simulink model "IEEE24bus"  (R2019b)
settings: Solver=VariableStepAuto  StartTime=0.0  StopTime=100  RelTol=1e-3
values from neighbouring files (symbols this model uses):
  C_b = 1/(w_b*Z_b)    (= 5.01433343075e-06)    [IEEE24_bus.m]
  Exc = [ 011	0	 200	0.02	1.12   0.5   0	0       0       0       0       0 ... (first row only)    [IEEE24_bus.m]
  G_data = [ 011	15.8 138	2.8	0.2     2.7	1.5     0.3     7.5     0.25	0.04	0.85	0.85	0.25	0.12	0 ... (first row only)    [IEEE24_bus.m]
  H011 = 4    [IEEE24_bus.m]
  H012 = 4    [IEEE24_bus.m]
  H013 = 4    [IEEE24_bus.m]
  H021 = 4    [IEEE24_bus.m]
  H022 = 4    [IEEE24_bus.m]
  H023 = 4    [IEEE24_bus.m]
  H024 = 4    [IEEE24_bus.m]
  H025 = 4    [IEEE24_bus.m]
  H026 = 4    [IEEE24_bus.m]
  H131 = 4    [IEEE24_bus.m]
  H132 = 4    [IEEE24_bus.m]
  H133 = 4    [IEEE24_bus.m]
  H134 = 4    [IEEE24_bus.m]
  H135 = 4    [IEEE24_bus.m]
  H151 = 4    [IEEE24_bus.m]
  H152 = 4    [IEEE24_bus.m]
  H153 = 4    [IEEE24_bus.m]
  H154 = 4    [IEEE24_bus.m]
  H161 = 4    [IEEE24_bus.m]
  H181 = 3.25    [IEEE24_bus.m]
  H211 = 4    [IEEE24_bus.m]
  H212 = 4    [IEEE24_bus.m]
  H213 = 4    [IEEE24_bus.m]
  H215 = 4    [IEEE24_bus.m]
  H216 = 4    [IEEE24_bus.m]
  H221 = 3.25    [IEEE24_bus.m]
  H231 = 4    [IEEE24_bus.m]
  H232 = 4    [IEEE24_bus.m]
  H233 = 4    [IEEE24_bus.m]
  H234 = 4    [IEEE24_bus.m]
  H235 = 4    [IEEE24_bus.m]
  L_b = Z_b/w_b    (= 1.40321608159)    [IEEE24_bus.m]
  PSSMODEL = 1    [IEEE24_bus.m]    (also in IEEE24bus_simplified_benchmark.m)
  Z_b = (V_b^2)/S_b    (= 529)    [IEEE24_bus.m]
undefined symbols (not defined in the file or in its folder): D1, Delta
libraries: powerlib x258, sps_avr x33, microgridLibrary x6
(part 3 of 6)

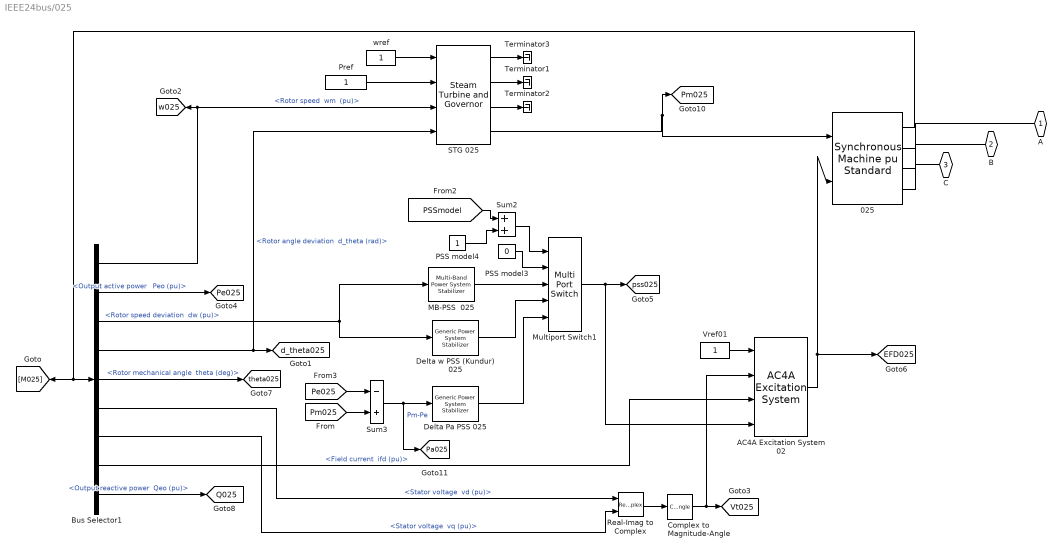
== system IEEE24bus/025 ==
  025 : powerlib/Machines/Synchronous Machine pu Standard  PresetModel=No  MechanicalLoad=Mechanical power Pm  ShowDetailedParameters=on  RotorType=Round  Units=per unit standard parameters  MeasurementBus=off  NominalParameters="[G_data(8,2)*1E6  G_data(8,3)*1E3  60]"  Reactances1=[G_data(8,6),G_data(8,8),G_data(8,10),G_data(8,7),G_data(8,12),G_data(8,14),G_data(8,5)]  Reactances2=[G_data(6,6),G_data(6,8),G_data(6,10),G_data(6,7),G_data(6,12),G_data(6,14),G_data(6,5)]  dAxisTimeConstants=Open-circuit  qAxisTimeConstants=Open-circuit  TimeConstants1="[G_data(6,9)  G_data(6,11)  G_data(6,13)  G_data(6,15)]"  TimeConstants2="[G_data(8,9)  G_data(8,11)  G_data(8,13)  G_data(8,15)]"  TimeConstants3="[  5.9  0.033  0.023  ]"  TimeConstants4=[ 8.0, 0.03, 0.3371, 0.0295 ]  TimeConstants5=[ 1.01, 0.053, 0.1 ]  TimeConstants6=[ 1.3201, 0.023, 1.0, 0.07 ]  TimeConstants7="[  1.01  0.053  0.051266  ]"  TimeConstants8=[ 1.3201, 0.0231, 0.3371, 0.0295 ]  StatorResistance=0  Mechanical="[ H025 0  4 ]"  PolePairs=4  InitialConditions=[0 -49.0871 0.832503 0.832503 0.832503 -10.6328 -130.633 109.367 2.39024]  SetSaturation=off  Saturation=[0.6404,0.7127,0.8441,0.9214,0.9956,1.082,1.19,1.316,1.457;0.7,0.7698,0.8872,0.9466,0.9969,1.046,1.1,1.151,1.201]  LoadFlowParameters=[1 3330000000 20000 0 0]  TsPowergui=0  TsBlock=-1  IterativeModel=Forward Euler  IterativeDiscreteModel=Trapezoidal non iterative  BusType=PV  Pref=G_data(8,2)*1e6  Qref=0  Qmin=-inf  Qmax=inf  PLF=0  QLF=0
      settings: SourceProductName=Simscape Power Systems
  AC4A Excitation System 02 : sps_avr/AC4A Excitation System  Tr=Exc(1,2)  KaTa="[Exc(1,3)   Exc(1,4)]"  VIminmax=[-10 10]  VRminmax=[-4.53 5.64]  TbTc="[Exc(1,5)  Exc(1,6)]"  Kc=0  v0=[1 2.3902]  TsBlock=0
      settings: SourceProductName=Simscape Power Systems  SourceProductBaseCode=PS
  Bus Selector1 : BusSelector  OutputSignals="Mechanical.Rotor speed  wm  (pu),Output active power   Peo (pu),Mechanical.Rotor speed deviation  dw (pu),Mechanical.Rotor angle deviation  d_theta (rad),Mechanical.Rotor mechanical angle  theta (deg),dq0 components.Stator voltage  vd (pu),dq0 components.Stator voltage  vq (pu),dq0 components.Field current  ifd (pu),Output reactive power  Qeo (pu)"
  Complex to Magnitude-Angle : ComplexToMagnitudeAngle  Output=Magnitude
  "Delta Pa PSS 025 " : powerlib/Machines/Generic Power System Stabilizer  Tsensor=15e-3  K=2.5*1.25  Twashout=1  Tleadlag1=[60e-3 1]  Tleadlag2=[0 0]  VSlimits=[-0.15 0.15]  Vinit=0  Plot_On=off  MagdB_On=on  FreqRange=logspace(-2,2,500)
      settings: SourceProductName=Simscape Power Systems  SourceProductBaseCode=PS
  "Delta w PSS (Kundur) 025 " : powerlib/Machines/Generic Power System Stabilizer  Tsensor=15e-3  K=30  Twashout=10  Tleadlag1=[50e-3 20e-3]  Tleadlag2=[3 5.4]  VSlimits=[-0.15 0.15]  Vinit=0  Plot_On=off  MagdB_On=on  FreqRange=logspace(-2,2,500)
      settings: SourceProductName=Simscape Power Systems  SourceProductBaseCode=PS
  MB-PSS  025 : powerlib/Machines/Multi-Band Power System Stabilizer  OperationMode=Simplified settings  Kg=1  GL=[0.1 10]  GI="[1  10]"  GH="[13  120]"  GLd=[66 66 9.4]  TcLF=[1.667 2 0 0 0 0 2 2.4 0 0 0 0 1 1]  GId=[66 66 47.6]  TcIF=[1 1 0.25 0.3 0 0 1 1 0.3 0.36 0 0 0 0]  GHd=[66 66 233]  TcHF="[0.01 0.012 0 0 0 0  0.012 0.0144 0 0 0 0 1 1]"  LIM=[.075 .15 .15 .15]  Plot_On=off  MagdB_On=off  FreqRange=logspace(-2,2,500)
      settings: SourceProductName=Simscape Power Systems  SourceProductBaseCode=PS
  Multiport Switch1 : MultiPortSwitch  Inputs=4  InputSameDT=on
  PSS model3 : Constant  Value=0
  PSS model4 : Constant
  Pref : Constant
  Real-Imag to Complex : RealImagToComplex
  STG 025 : powerlib/Machines/Steam Turbine and Governor  gentype=Tandem-compound (single mass)  reg1="[ 1  0.05    0 ]"  reg2="[ 0.001  0.15 ]"  reg3="[ -0.1  0.1  0  4.496 ]"  N=3600  turb1="[ 0  10   3.3   0.5   ]"  turb2="[   0   0.36    0.36   0.28   ]"  HA="[ 0.046  1.430  1.465   0.192 ]"  KA="[ 90.44  53.88  64.59   62.94  ]"  DA="[ 0.0115  0.3575  0.3663   0.0137  ]"  ini1=1  ini2=[0.779316,-31.4247]
      settings: SourceProductName=Simscape Power Systems  SourceProductBaseCode=PS
  Sum2 : Sum  SaturateOnIntegerOverflow=on  InputSameDT=on  OutDataTypeStr=Inherit: Same as first input
  Sum3 : Sum  Inputs=-+  SaturateOnIntegerOverflow=on  InputSameDT=on  OutDataTypeStr=Inherit: Same as first input
  Terminator1 : Terminator
  Terminator2 : Terminator
  Terminator3 : Terminator
  Vref01 : Constant
  wref : Constant
  A : PMIOPort  Side=Left
  B : PMIOPort  Port=2  Side=Left
  C : PMIOPort  Port=3  Side=Left
  tag scope: EFD025=global, Pa025=global, Pe025=global, Pm025=global, Q025=global, Vt025=global, d_theta025=global, pss025=global, theta025=global, w025=global
  wires:
  Bus Selector1/7 -> Real-Imag to Complex/2  "<Stator voltage  vq (pu)>"
  Bus Selector1/6 -> Real-Imag to Complex/1  "<Stator voltage  vd (pu)>"
  wref/1 -> STG 025/1
  Vref01/1 -> AC4A Excitation System 02/1
  Bus Selector1/4 -> [d_theta025], STG 025/4  "<Rotor angle deviation  d_theta (rad)>"
  025/1 -> Bus Selector1/1, [M025]
  Bus Selector1/1 -> [w025], STG 025/3  "<Rotor speed  wm  (pu)>"
  Bus Selector1/3 -> "Delta w PSS (Kundur) 025 "/1, MB-PSS  025/1  "<Rotor speed deviation  dw (pu)>"
  Real-Imag to Complex/1 -> Complex to Magnitude-Angle/1
  Complex to Magnitude-Angle/1 -> AC4A Excitation System 02/2, [Vt025]
  AC4A Excitation System 02/1 -> 025/2, [EFD025]
  Multiport Switch1/1 -> AC4A Excitation System 02/4, [pss025]
  Bus Selector1/5 -> [theta025]  "<Rotor mechanical angle  theta (deg)>"
  Bus Selector1/2 -> [Pe025]  "<Output active power   Peo (pu)>"
  Bus Selector1/8 -> AC4A Excitation System 02/3  "<Field current  ifd (pu)>"
  STG 025/4 -> [Pm025], 025/1
  Pref/1 -> STG 025/2
  Bus Selector1/9 -> [Q025]  "<Output reactive power  Qeo (pu)>"
  PSS model4/1 -> Sum2/2
  Sum2/1 -> Multiport Switch1/1
  [PSSmodel] -> Sum2/1
  PSS model3/1 -> Multiport Switch1/2
  Sum3/1 -> [Pa025], "Delta Pa PSS 025 "/1  "Pm-Pe"
  "Delta Pa PSS 025 "/1 -> Multiport Switch1/5
  "Delta w PSS (Kundur) 025 "/1 -> Multiport Switch1/4
  [Pm025] -> Sum3/2
  [Pe025] -> Sum3/1
  MB-PSS  025/1 -> Multiport Switch1/3
  STG 025/1 -> Terminator3/1
  STG 025/2 -> Terminator1/1
  STG 025/3 -> Terminator2/1
  connections:
  025/RConn1 -- A/RConn1
  025/RConn2 -- B/RConn1
  025/RConn3 -- C/RConn1

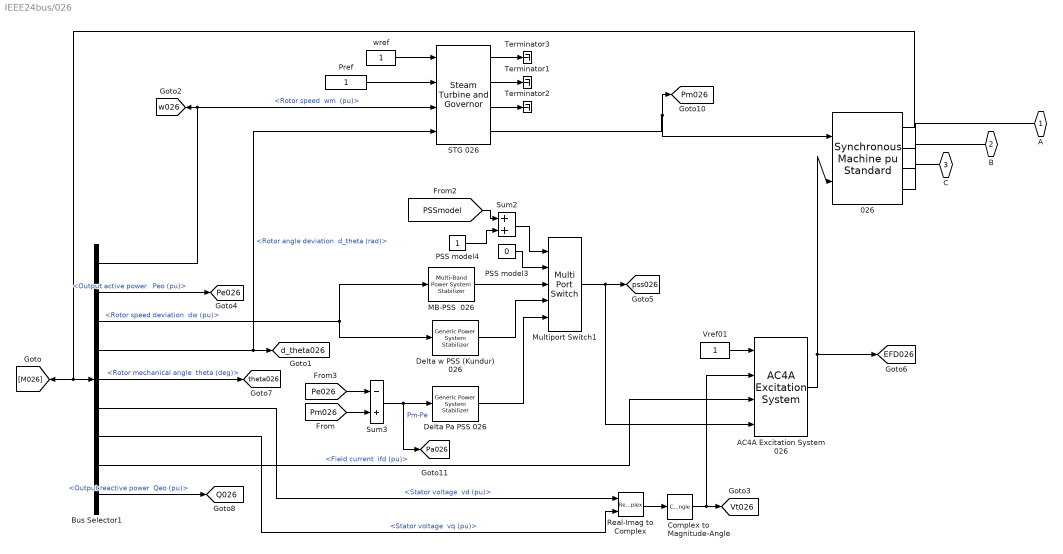
== system IEEE24bus/026 ==
  026 : powerlib/Machines/Synchronous Machine pu Standard  PresetModel=No  MechanicalLoad=Mechanical power Pm  ShowDetailedParameters=on  RotorType=Round  Units=per unit standard parameters  MeasurementBus=off  NominalParameters="[G_data(9,2)*1E6  G_data(9,3)*1E3  60]"  Reactances1=[G_data(9,6),G_data(9,8),G_data(9,10),G_data(9,7),G_data(9,12),G_data(9,14),G_data(9,5)]  Reactances2=[G_data(6,6),G_data(6,8),G_data(6,10),G_data(6,7),G_data(6,12),G_data(6,14),G_data(6,5)]  dAxisTimeConstants=Open-circuit  qAxisTimeConstants=Open-circuit  TimeConstants1="[G_data(6,9)  G_data(6,11)  G_data(6,13)  G_data(6,15)]"  TimeConstants2="[G_data(9,9)  G_data(9,11)  G_data(9,13)  G_data(9,15)]"  TimeConstants3="[  5.9  0.033  0.023  ]"  TimeConstants4=[ 8.0, 0.03, 0.3371, 0.0295 ]  TimeConstants5=[ 1.01, 0.053, 0.1 ]  TimeConstants6=[ 1.3201, 0.023, 1.0, 0.07 ]  TimeConstants7="[  1.01  0.053  0.051266  ]"  TimeConstants8=[ 1.3201, 0.0231, 0.3371, 0.0295 ]  StatorResistance=0  Mechanical="[ H026 0  4 ]"  PolePairs=4  InitialConditions=[0 -49.0871 0.832503 0.832503 0.832503 -10.6328 -130.633 109.367 2.39024]  SetSaturation=off  Saturation=[0.6404,0.7127,0.8441,0.9214,0.9956,1.082,1.19,1.316,1.457;0.7,0.7698,0.8872,0.9466,0.9969,1.046,1.1,1.151,1.201]  LoadFlowParameters=[1 3330000000 20000 0 0]  TsPowergui=0  TsBlock=-1  IterativeModel=Forward Euler  IterativeDiscreteModel=Trapezoidal non iterative  BusType=PV  Pref=G_data(9,2)*1e6  Qref=0  Qmin=-inf  Qmax=inf  PLF=0  QLF=0
      settings: SourceProductName=Simscape Power Systems
  AC4A Excitation System 026 : sps_avr/AC4A Excitation System  Tr=Exc(1,2)  KaTa="[Exc(1,3)   Exc(1,4)]"  VIminmax=[-10 10]  VRminmax=[-4.53 5.64]  TbTc="[Exc(1,5)  Exc(1,6)]"  Kc=0  v0=[1 2.3902]  TsBlock=0
      settings: SourceProductName=Simscape Power Systems  SourceProductBaseCode=PS
  Bus Selector1 : BusSelector  OutputSignals="Mechanical.Rotor speed  wm  (pu),Output active power   Peo (pu),Mechanical.Rotor speed deviation  dw (pu),Mechanical.Rotor angle deviation  d_theta (rad),Mechanical.Rotor mechanical angle  theta (deg),dq0 components.Stator voltage  vd (pu),dq0 components.Stator voltage  vq (pu),dq0 components.Field current  ifd (pu),Output reactive power  Qeo (pu)"
  Complex to Magnitude-Angle : ComplexToMagnitudeAngle  Output=Magnitude
  "Delta Pa PSS 026 " : powerlib/Machines/Generic Power System Stabilizer  Tsensor=15e-3  K=2.5*1.25  Twashout=1  Tleadlag1=[60e-3 1]  Tleadlag2=[0 0]  VSlimits=[-0.15 0.15]  Vinit=0  Plot_On=off  MagdB_On=on  FreqRange=logspace(-2,2,500)
      settings: SourceProductName=Simscape Power Systems  SourceProductBaseCode=PS
  "Delta w PSS (Kundur) 026 " : powerlib/Machines/Generic Power System Stabilizer  Tsensor=15e-3  K=30  Twashout=10  Tleadlag1=[50e-3 20e-3]  Tleadlag2=[3 5.4]  VSlimits=[-0.15 0.15]  Vinit=0  Plot_On=off  MagdB_On=on  FreqRange=logspace(-2,2,500)
      settings: SourceProductName=Simscape Power Systems  SourceProductBaseCode=PS
  MB-PSS  026 : powerlib/Machines/Multi-Band Power System Stabilizer  OperationMode=Simplified settings  Kg=1  GL=[0.1 10]  GI="[1  10]"  GH="[13  120]"  GLd=[66 66 9.4]  TcLF=[1.667 2 0 0 0 0 2 2.4 0 0 0 0 1 1]  GId=[66 66 47.6]  TcIF=[1 1 0.25 0.3 0 0 1 1 0.3 0.36 0 0 0 0]  GHd=[66 66 233]  TcHF="[0.01 0.012 0 0 0 0  0.012 0.0144 0 0 0 0 1 1]"  LIM=[.075 .15 .15 .15]  Plot_On=off  MagdB_On=off  FreqRange=logspace(-2,2,500)
      settings: SourceProductName=Simscape Power Systems  SourceProductBaseCode=PS
  Multiport Switch1 : MultiPortSwitch  Inputs=4  InputSameDT=on
  PSS model3 : Constant  Value=0
  PSS model4 : Constant
  Pref : Constant
  Real-Imag to Complex : RealImagToComplex
  STG 026 : powerlib/Machines/Steam Turbine and Governor  gentype=Tandem-compound (single mass)  reg1="[ 1  0.05    0 ]"  reg2="[ 0.001  0.15 ]"  reg3="[ -0.1  0.1  0  4.496 ]"  N=3600  turb1="[ 0  10   3.3   0.5   ]"  turb2="[   0   0.36    0.36   0.28   ]"  HA="[ 0.046  1.430  1.465   0.192 ]"  KA="[ 90.44  53.88  64.59   62.94  ]"  DA="[ 0.0115  0.3575  0.3663   0.0137  ]"  ini1=0.9  ini2=[0.779316,-31.4247]
      settings: SourceProductName=Simscape Power Systems  SourceProductBaseCode=PS
  Sum2 : Sum  SaturateOnIntegerOverflow=on  InputSameDT=on  OutDataTypeStr=Inherit: Same as first input
  Sum3 : Sum  Inputs=-+  SaturateOnIntegerOverflow=on  InputSameDT=on  OutDataTypeStr=Inherit: Same as first input
  Terminator1 : Terminator
  Terminator2 : Terminator
  Terminator3 : Terminator
  Vref01 : Constant
  wref : Constant
  A : PMIOPort  Side=Left
  B : PMIOPort  Port=2  Side=Left
  C : PMIOPort  Port=3  Side=Left
  tag scope: EFD026=global, Pa026=global, Pe026=global, Pm026=global, Q026=global, Vt026=global, d_theta026=global, pss026=global, theta026=global, w026=global
  wires:
  Bus Selector1/7 -> Real-Imag to Complex/2  "<Stator voltage  vq (pu)>"
  Bus Selector1/6 -> Real-Imag to Complex/1  "<Stator voltage  vd (pu)>"
  wref/1 -> STG 026/1
  Vref01/1 -> AC4A Excitation System 026/1
  Bus Selector1/4 -> [d_theta026], STG 026/4  "<Rotor angle deviation  d_theta (rad)>"
  026/1 -> Bus Selector1/1, [M026]
  Bus Selector1/1 -> [w026], STG 026/3  "<Rotor speed  wm  (pu)>"
  Bus Selector1/3 -> "Delta w PSS (Kundur) 026 "/1, MB-PSS  026/1  "<Rotor speed deviation  dw (pu)>"
  Real-Imag to Complex/1 -> Complex to Magnitude-Angle/1
  Complex to Magnitude-Angle/1 -> AC4A Excitation System 026/2, [Vt026]
  AC4A Excitation System 026/1 -> 026/2, [EFD026]
  Multiport Switch1/1 -> AC4A Excitation System 026/4, [pss026]
  Bus Selector1/5 -> [theta026]  "<Rotor mechanical angle  theta (deg)>"
  Bus Selector1/2 -> [Pe026]  "<Output active power   Peo (pu)>"
  Bus Selector1/8 -> AC4A Excitation System 026/3  "<Field current  ifd (pu)>"
  STG 026/4 -> [Pm026], 026/1
  Pref/1 -> STG 026/2
  Bus Selector1/9 -> [Q026]  "<Output reactive power  Qeo (pu)>"
  PSS model4/1 -> Sum2/2
  Sum2/1 -> Multiport Switch1/1
  [PSSmodel] -> Sum2/1
  PSS model3/1 -> Multiport Switch1/2
  Sum3/1 -> [Pa026], "Delta Pa PSS 026 "/1  "Pm-Pe"
  "Delta Pa PSS 026 "/1 -> Multiport Switch1/5
  "Delta w PSS (Kundur) 026 "/1 -> Multiport Switch1/4
  [Pm026] -> Sum3/2
  [Pe026] -> Sum3/1
  MB-PSS  026/1 -> Multiport Switch1/3
  STG 026/1 -> Terminator3/1
  STG 026/2 -> Terminator1/1
  STG 026/3 -> Terminator2/1
  connections:
  026/RConn1 -- A/RConn1
  026/RConn2 -- B/RConn1
  026/RConn3 -- C/RConn1

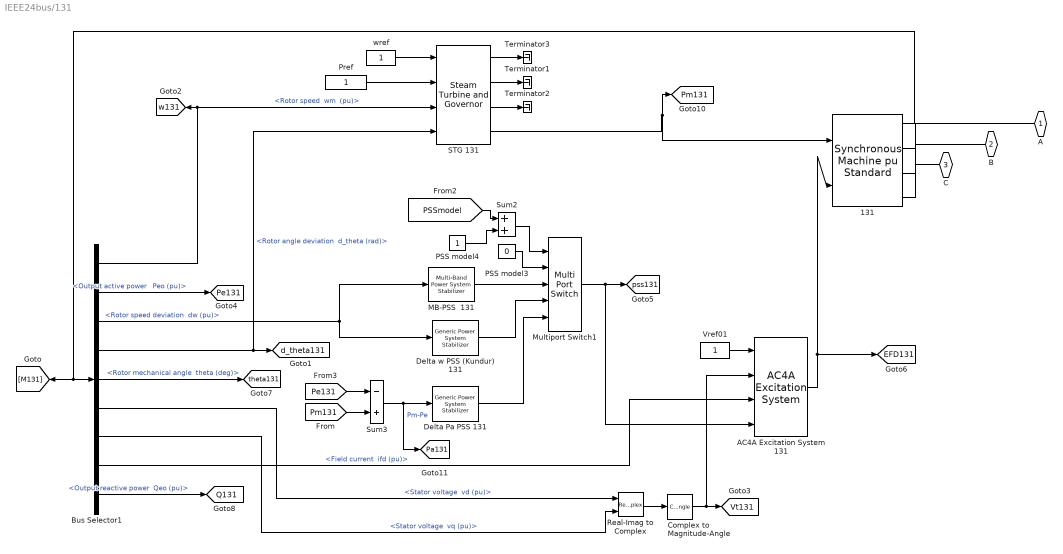
== system IEEE24bus/131 ==
  131 : powerlib/Machines/Synchronous Machine pu Standard  PresetModel=No  MechanicalLoad=Mechanical power Pm  ShowDetailedParameters=on  RotorType=Round  Units=per unit standard parameters  MeasurementBus=off  NominalParameters="[165*1E6  G_data(11,3)*1E3  60]"  Reactances1=[G_data(11,6),G_data(11,8),G_data(11,10),G_data(11,7),G_data(11,12),G_data(11,14),G_data(11,5)]  Reactances2=[G_data(6,6),G_data(6,8),G_data(6,10),G_data(6,7),G_data(6,12),G_data(6,14),G_data(6,5)]  dAxisTimeConstants=Open-circuit  qAxisTimeConstants=Open-circuit  TimeConstants1="[G_data(6,9)  G_data(6,11)  G_data(6,13)  G_data(6,15)]"  TimeConstants2="[G_data(11,9)  G_data(11,11)  G_data(11,13)  G_data(11,15)]"  TimeConstants3="[  5.9  0.033  0.023  ]"  TimeConstants4=[ 8.0, 0.03, 0.3371, 0.0295 ]  TimeConstants5=[ 1.01, 0.053, 0.1 ]  TimeConstants6=[ 1.3201, 0.023, 1.0, 0.07 ]  TimeConstants7="[  1.01  0.053  0.051266  ]"  TimeConstants8=[ 1.3201, 0.0231, 0.3371, 0.0295 ]  StatorResistance=0  Mechanical="[ H131 0  4 ]"  PolePairs=4  InitialConditions=[0 -49.0871 0.832503 0.832503 0.832503 -10.6328 -130.633 109.367 2.39024]  SetSaturation=off  Saturation=[0.6404,0.7127,0.8441,0.9214,0.9956,1.082,1.19,1.316,1.457;0.7,0.7698,0.8872,0.9466,0.9969,1.046,1.1,1.151,1.201]  LoadFlowParameters=[1 3330000000 20000 0 0]  TsPowergui=0  TsBlock=-1  IterativeModel=Forward Euler  IterativeDiscreteModel=Trapezoidal non iterative  BusType=PV  Pref=G_data(11,2)*1e6  Qref=0  Qmin=-inf  Qmax=inf  PLF=0  QLF=0
      settings: SourceProductName=Simscape Power Systems
  AC4A Excitation System 131 : sps_avr/AC4A Excitation System  Tr=Exc(11,2)  KaTa="[Exc(11,3)   Exc(11,4)]"  VIminmax=[-10 10]  VRminmax=[-4.53 5.64]  TbTc="[Exc(11,5)  Exc(11,6)]"  Kc=0  v0=[1 2.3902]  TsBlock=0
      settings: SourceProductName=Simscape Power Systems  SourceProductBaseCode=PS
  Bus Selector1 : BusSelector  OutputSignals="Mechanical.Rotor speed  wm  (pu),Output active power   Peo (pu),Mechanical.Rotor speed deviation  dw (pu),Mechanical.Rotor angle deviation  d_theta (rad),Mechanical.Rotor mechanical angle  theta (deg),dq0 components.Stator voltage  vd (pu),dq0 components.Stator voltage  vq (pu),dq0 components.Field current  ifd (pu),Output reactive power  Qeo (pu)"
  Complex to Magnitude-Angle : ComplexToMagnitudeAngle  Output=Magnitude
  Delta Pa PSS 131 : powerlib/Machines/Generic Power System Stabilizer  Tsensor=15e-3  K=2.5*1.25  Twashout=1  Tleadlag1=[60e-3 1]  Tleadlag2=[0 0]  VSlimits=[-0.15 0.15]  Vinit=0  Plot_On=off  MagdB_On=on  FreqRange=logspace(-2,2,500)
      settings: SourceProductName=Simscape Power Systems  SourceProductBaseCode=PS
  "Delta w PSS (Kundur) 131 " : powerlib/Machines/Generic Power System Stabilizer  Tsensor=15e-3  K=30  Twashout=10  Tleadlag1=[50e-3 20e-3]  Tleadlag2=[3 5.4]  VSlimits=[-0.15 0.15]  Vinit=0  Plot_On=off  MagdB_On=on  FreqRange=logspace(-2,2,500)
      settings: SourceProductName=Simscape Power Systems  SourceProductBaseCode=PS
  MB-PSS  131 : powerlib/Machines/Multi-Band Power System Stabilizer  OperationMode=Simplified settings  Kg=1  GL=[0.1 10]  GI="[1  10]"  GH="[13  120]"  GLd=[66 66 9.4]  TcLF=[1.667 2 0 0 0 0 2 2.4 0 0 0 0 1 1]  GId=[66 66 47.6]  TcIF=[1 1 0.25 0.3 0 0 1 1 0.3 0.36 0 0 0 0]  GHd=[66 66 233]  TcHF="[0.01 0.012 0 0 0 0  0.012 0.0144 0 0 0 0 1 1]"  LIM=[.075 .15 .15 .15]  Plot_On=off  MagdB_On=off  FreqRange=logspace(-2,2,500)
      settings: SourceProductName=Simscape Power Systems  SourceProductBaseCode=PS
  Multiport Switch1 : MultiPortSwitch  Inputs=4  InputSameDT=on
  PSS model3 : Constant  Value=0
  PSS model4 : Constant
  Pref : Constant
  Real-Imag to Complex : RealImagToComplex
  STG 131 : powerlib/Machines/Steam Turbine and Governor  gentype=Tandem-compound (single mass)  reg1="[ 1  0.05    0 ]"  reg2="[ 0.001  0.15 ]"  reg3="[ -0.1  0.1  0  4.496 ]"  N=3600  turb1="[ 0  10   3.3   0.5   ]"  turb2="[   0   0.36    0.36   0.28   ]"  HA="[ 0.046  1.430  1.465   0.192 ]"  KA="[ 90.44  53.88  64.59   62.94  ]"  DA="[ 0.0115  0.3575  0.3663   0.0137  ]"  ini1=0.98  ini2=[0.779316,-31.4247]
      settings: SourceProductName=Simscape Power Systems  SourceProductBaseCode=PS
  Sum2 : Sum  SaturateOnIntegerOverflow=on  InputSameDT=on  OutDataTypeStr=Inherit: Same as first input
  Sum3 : Sum  Inputs=-+  SaturateOnIntegerOverflow=on  InputSameDT=on  OutDataTypeStr=Inherit: Same as first input
  Terminator1 : Terminator
  Terminator2 : Terminator
  Terminator3 : Terminator
  Vref01 : Constant
  wref : Constant
  A : PMIOPort  Side=Left
  B : PMIOPort  Port=2  Side=Left
  C : PMIOPort  Port=3  Side=Left
  tag scope: EFD131=global, Pa131=global, Pe131=global, Pm131=global, Q131=global, Vt131=global, d_theta131=global, pss131=global, theta131=global, w131=global
  wires:
  Bus Selector1/7 -> Real-Imag to Complex/2  "<Stator voltage  vq (pu)>"
  Bus Selector1/6 -> Real-Imag to Complex/1  "<Stator voltage  vd (pu)>"
  wref/1 -> STG 131/1
  Vref01/1 -> AC4A Excitation System 131/1
  Bus Selector1/4 -> [d_theta131], STG 131/4  "<Rotor angle deviation  d_theta (rad)>"
  131/1 -> Bus Selector1/1, [M131]
  Bus Selector1/1 -> [w131], STG 131/3  "<Rotor speed  wm  (pu)>"
  Bus Selector1/3 -> "Delta w PSS (Kundur) 131 "/1, MB-PSS  131/1  "<Rotor speed deviation  dw (pu)>"
  Real-Imag to Complex/1 -> Complex to Magnitude-Angle/1
  Complex to Magnitude-Angle/1 -> AC4A Excitation System 131/2, [Vt131]
  AC4A Excitation System 131/1 -> 131/2, [EFD131]
  Multiport Switch1/1 -> AC4A Excitation System 131/4, [pss131]
  Bus Selector1/5 -> [theta131]  "<Rotor mechanical angle  theta (deg)>"
  Bus Selector1/2 -> [Pe131]  "<Output active power   Peo (pu)>"
  Bus Selector1/8 -> AC4A Excitation System 131/3  "<Field current  ifd (pu)>"
  STG 131/4 -> [Pm131], 131/1
  Pref/1 -> STG 131/2
  Bus Selector1/9 -> [Q131]  "<Output reactive power  Qeo (pu)>"
  PSS model4/1 -> Sum2/2
  Sum2/1 -> Multiport Switch1/1
  [PSSmodel] -> Sum2/1
  PSS model3/1 -> Multiport Switch1/2
  Sum3/1 -> [Pa131], Delta Pa PSS 131/1  "Pm-Pe"
  Delta Pa PSS 131/1 -> Multiport Switch1/5
  "Delta w PSS (Kundur) 131 "/1 -> Multiport Switch1/4
  [Pm131] -> Sum3/2
  [Pe131] -> Sum3/1
  MB-PSS  131/1 -> Multiport Switch1/3
  STG 131/1 -> Terminator3/1
  STG 131/2 -> Terminator1/1
  STG 131/3 -> Terminator2/1
  connections:
  131/RConn1 -- A/RConn1
  131/RConn2 -- B/RConn1
  131/RConn3 -- C/RConn1

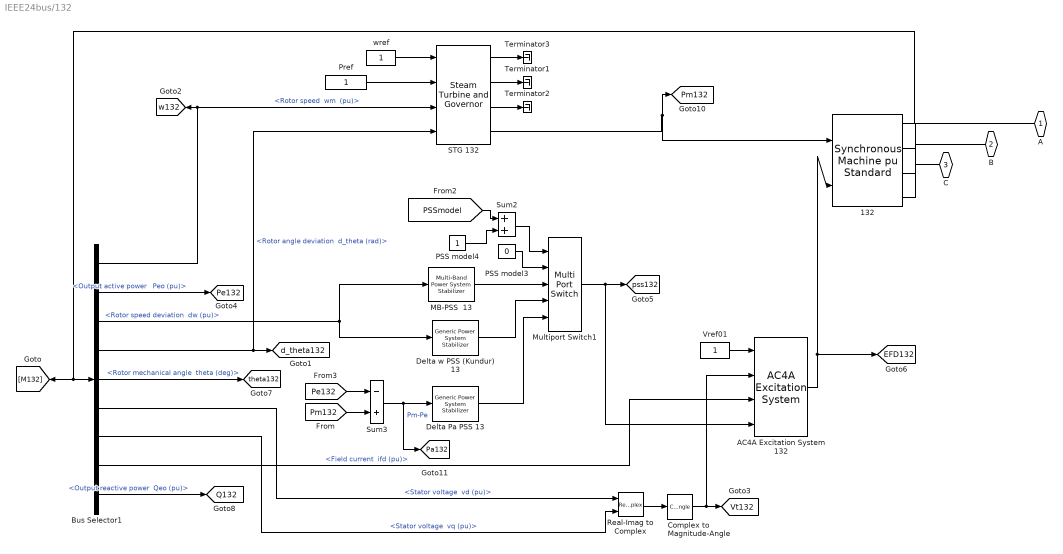
== system IEEE24bus/132 ==
  132 : powerlib/Machines/Synchronous Machine pu Standard  PresetModel=No  MechanicalLoad=Mechanical power Pm  ShowDetailedParameters=on  RotorType=Round  Units=per unit standard parameters  MeasurementBus=off  NominalParameters="[200*1E6  G_data(12,3)*1E3  60]"  Reactances1=[G_data(12,6),G_data(12,8),G_data(12,10),G_data(12,7),G_data(12,12),G_data(12,14),G_data(12,5)]  Reactances2=[G_data(6,6),G_data(6,8),G_data(6,10),G_data(6,7),G_data(6,12),G_data(6,14),G_data(6,5)]  dAxisTimeConstants=Open-circuit  qAxisTimeConstants=Open-circuit  TimeConstants1="[G_data(6,9)  G_data(6,11)  G_data(6,13)  G_data(6,15)]"  TimeConstants2="[G_data(12,9)  G_data(12,11)  G_data(12,13)  G_data(12,15)]"  TimeConstants3="[  5.9  0.033  0.023  ]"  TimeConstants4=[ 8.0, 0.03, 0.3371, 0.0295 ]  TimeConstants5=[ 1.01, 0.053, 0.1 ]  TimeConstants6=[ 1.3201, 0.023, 1.0, 0.07 ]  TimeConstants7="[  1.01  0.053  0.051266  ]"  TimeConstants8=[ 1.3201, 0.0231, 0.3371, 0.0295 ]  StatorResistance=0  Mechanical="[ H132 0  4 ]"  PolePairs=4  InitialConditions=[0 -49.0871 0.832503 0.832503 0.832503 -10.6328 -130.633 109.367 2.39024]  SetSaturation=off  Saturation=[0.6404,0.7127,0.8441,0.9214,0.9956,1.082,1.19,1.316,1.457;0.7,0.7698,0.8872,0.9466,0.9969,1.046,1.1,1.151,1.201]  LoadFlowParameters=[1 3330000000 20000 0 0]  TsPowergui=0  TsBlock=-1  IterativeModel=Forward Euler  IterativeDiscreteModel=Trapezoidal non iterative  BusType=PV  Pref=200*1e6  Qref=0  Qmin=-inf  Qmax=inf  PLF=0  QLF=0
      settings: SourceProductName=Simscape Power Systems
  AC4A Excitation System 132 : sps_avr/AC4A Excitation System  Tr=Exc(12,2)  KaTa="[Exc(12,3)   Exc(12,4)]"  VIminmax=[-10 10]  VRminmax=[-4.53 5.64]  TbTc="[Exc(12,5)  Exc(12,6)]"  Kc=0  v0=[1 2.3902]  TsBlock=0
      settings: SourceProductName=Simscape Power Systems  SourceProductBaseCode=PS
  Bus Selector1 : BusSelector  OutputSignals="Mechanical.Rotor speed  wm  (pu),Output active power   Peo (pu),Mechanical.Rotor speed deviation  dw (pu),Mechanical.Rotor angle deviation  d_theta (rad),Mechanical.Rotor mechanical angle  theta (deg),dq0 components.Stator voltage  vd (pu),dq0 components.Stator voltage  vq (pu),dq0 components.Field current  ifd (pu),Output reactive power  Qeo (pu)"
  Complex to Magnitude-Angle : ComplexToMagnitudeAngle  Output=Magnitude
  "Delta Pa PSS 13 " : powerlib/Machines/Generic Power System Stabilizer  Tsensor=15e-3  K=2.5*1.25  Twashout=1  Tleadlag1=[60e-3 1]  Tleadlag2=[0 0]  VSlimits=[-0.15 0.15]  Vinit=0  Plot_On=off  MagdB_On=on  FreqRange=logspace(-2,2,500)
      settings: SourceProductName=Simscape Power Systems  SourceProductBaseCode=PS
  "Delta w PSS (Kundur) 13 " : powerlib/Machines/Generic Power System Stabilizer  Tsensor=15e-3  K=30  Twashout=10  Tleadlag1=[50e-3 20e-3]  Tleadlag2=[3 5.4]  VSlimits=[-0.15 0.15]  Vinit=0  Plot_On=off  MagdB_On=on  FreqRange=logspace(-2,2,500)
      settings: SourceProductName=Simscape Power Systems  SourceProductBaseCode=PS
  MB-PSS  13 : powerlib/Machines/Multi-Band Power System Stabilizer  OperationMode=Simplified settings  Kg=1  GL=[0.1 10]  GI="[1  10]"  GH="[13  120]"  GLd=[66 66 9.4]  TcLF=[1.667 2 0 0 0 0 2 2.4 0 0 0 0 1 1]  GId=[66 66 47.6]  TcIF=[1 1 0.25 0.3 0 0 1 1 0.3 0.36 0 0 0 0]  GHd=[66 66 233]  TcHF="[0.01 0.012 0 0 0 0  0.012 0.0144 0 0 0 0 1 1]"  LIM=[.075 .15 .15 .15]  Plot_On=off  MagdB_On=off  FreqRange=logspace(-2,2,500)
      settings: SourceProductName=Simscape Power Systems  SourceProductBaseCode=PS
  Multiport Switch1 : MultiPortSwitch  Inputs=4  InputSameDT=on
  PSS model3 : Constant  Value=0
  PSS model4 : Constant
  Pref : Constant
  Real-Imag to Complex : RealImagToComplex
  STG 132 : powerlib/Machines/Steam Turbine and Governor  gentype=Tandem-compound (single mass)  reg1="[ 1  0.05    0 ]"  reg2="[ 0.001  0.15 ]"  reg3="[ -0.1  0.1  0  4.496 ]"  N=3600  turb1="[ 0  10   3.3   0.5   ]"  turb2="[   0   0.36    0.36   0.28   ]"  HA="[ 0.046  1.430  1.465   0.192 ]"  KA="[ 90.44  53.88  64.59   62.94  ]"  DA="[ 0.0115  0.3575  0.3663   0.0137  ]"  ini1=0.975  ini2=[0.779316,-31.4247]
      settings: SourceProductName=Simscape Power Systems  SourceProductBaseCode=PS
  Sum2 : Sum  SaturateOnIntegerOverflow=on  InputSameDT=on  OutDataTypeStr=Inherit: Same as first input
  Sum3 : Sum  Inputs=-+  SaturateOnIntegerOverflow=on  InputSameDT=on  OutDataTypeStr=Inherit: Same as first input
  Terminator1 : Terminator
  Terminator2 : Terminator
  Terminator3 : Terminator
  Vref01 : Constant
  wref : Constant
  A : PMIOPort  Side=Left
  B : PMIOPort  Port=2  Side=Left
  C : PMIOPort  Port=3  Side=Left
  tag scope: EFD132=global, Pa132=global, Pe132=global, Pm132=global, Q132=global, Vt132=global, d_theta132=global, pss132=global, theta132=global, w132=global
  wires:
  Bus Selector1/7 -> Real-Imag to Complex/2  "<Stator voltage  vq (pu)>"
  Bus Selector1/6 -> Real-Imag to Complex/1  "<Stator voltage  vd (pu)>"
  wref/1 -> STG 132/1
  Vref01/1 -> AC4A Excitation System 132/1
  Bus Selector1/4 -> [d_theta132], STG 132/4  "<Rotor angle deviation  d_theta (rad)>"
  132/1 -> Bus Selector1/1, [M132]
  Bus Selector1/1 -> [w132], STG 132/3  "<Rotor speed  wm  (pu)>"
  Bus Selector1/3 -> "Delta w PSS (Kundur) 13 "/1, MB-PSS  13/1  "<Rotor speed deviation  dw (pu)>"
  Real-Imag to Complex/1 -> Complex to Magnitude-Angle/1
  Complex to Magnitude-Angle/1 -> AC4A Excitation System 132/2, [Vt132]
  AC4A Excitation System 132/1 -> 132/2, [EFD132]
  Multiport Switch1/1 -> AC4A Excitation System 132/4, [pss132]
  Bus Selector1/5 -> [theta132]  "<Rotor mechanical angle  theta (deg)>"
  Bus Selector1/2 -> [Pe132]  "<Output active power   Peo (pu)>"
  Bus Selector1/8 -> AC4A Excitation System 132/3  "<Field current  ifd (pu)>"
  STG 132/4 -> [Pm132], 132/1
  Pref/1 -> STG 132/2
  Bus Selector1/9 -> [Q132]  "<Output reactive power  Qeo (pu)>"
  PSS model4/1 -> Sum2/2
  Sum2/1 -> Multiport Switch1/1
  [PSSmodel] -> Sum2/1
  PSS model3/1 -> Multiport Switch1/2
  Sum3/1 -> [Pa132], "Delta Pa PSS 13 "/1  "Pm-Pe"
  "Delta Pa PSS 13 "/1 -> Multiport Switch1/5
  "Delta w PSS (Kundur) 13 "/1 -> Multiport Switch1/4
  [Pm132] -> Sum3/2
  [Pe132] -> Sum3/1
  MB-PSS  13/1 -> Multiport Switch1/3
  STG 132/1 -> Terminator3/1
  STG 132/2 -> Terminator1/1
  STG 132/3 -> Terminator2/1
  connections:
  132/RConn1 -- A/RConn1
  132/RConn2 -- B/RConn1
  132/RConn3 -- C/RConn1

== system IEEE24bus/133 ==
  133 : powerlib/Machines/Synchronous Machine pu Standard  PresetModel=No  MechanicalLoad=Mechanical power Pm  ShowDetailedParameters=on  RotorType=Round  Units=per unit standard parameters  MeasurementBus=off  NominalParameters="[G_data(13,2)*1E6  G_data(13,3)*1E3  60]"  Reactances1=[G_data(13,6),G_data(13,8),G_data(13,10),G_data(13,7),G_data(13,12),G_data(13,14),G_data(13,5)]  Reactances2=[G_data(6,6),G_data(6,8),G_data(6,10),G_data(6,7),G_data(6,12),G_data(6,14),G_data(6,5)]  dAxisTimeConstants=Open-circuit  qAxisTimeConstants=Open-circuit  TimeConstants1="[G_data(6,9)  G_data(6,11)  G_data(6,13)  G_data(6,15)]"  TimeConstants2="[G_data(13,9)  G_data(13,11)  G_data(13,13)  G_data(13,15)]"  TimeConstants3="[  5.9  0.033  0.023  ]"  TimeConstants4=[ 8.0, 0.03, 0.3371, 0.0295 ]  TimeConstants5=[ 1.01, 0.053, 0.1 ]  TimeConstants6=[ 1.3201, 0.023, 1.0, 0.07 ]  TimeConstants7="[  1.01  0.053  0.051266  ]"  TimeConstants8=[ 1.3201, 0.0231, 0.3371, 0.0295 ]  StatorResistance=0  Mechanical="[ H133 0  4 ]"  PolePairs=4  InitialConditions=[0 -49.0871 0.832503 0.832503 0.832503 -10.6328 -130.633 109.367 2.39024]  SetSaturation=off  Saturation=[0.6404,0.7127,0.8441,0.9214,0.9956,1.082,1.19,1.316,1.457;0.7,0.7698,0.8872,0.9466,0.9969,1.046,1.1,1.151,1.201]  LoadFlowParameters=[1 3330000000 20000 0 0]  TsPowergui=0  TsBlock=-1  IterativeModel=Forward Euler  IterativeDiscreteModel=Trapezoidal non iterative  BusType=PV  Pref=G_data(13,2)*1e6  Qref=0  Qmin=-inf  Qmax=inf  PLF=0  QLF=0
      settings: SourceProductName=Simscape Power Systems
  AC4A Excitation System 133 : sps_avr/AC4A Excitation System  Tr=Exc(13,2)  KaTa="[Exc(13,3)   Exc(13,4)]"  VIminmax=[-10 10]  VRminmax=[-4.53 5.64]  TbTc="[Exc(13,5)  Exc(13,6)]"  Kc=0  v0=[1 2.3902]  TsBlock=0
      settings: SourceProductName=Simscape Power Systems  SourceProductBaseCode=PS
  Bus Selector1 : BusSelector  OutputSignals="Mechanical.Rotor speed  wm  (pu),Output active power   Peo (pu),Mechanical.Rotor speed deviation  dw (pu),Mechanical.Rotor angle deviation  d_theta (rad),Mechanical.Rotor mechanical angle  theta (deg),dq0 components.Stator voltage  vd (pu),dq0 components.Stator voltage  vq (pu),dq0 components.Field current  ifd (pu),Output reactive power  Qeo (pu)"
  Complex to Magnitude-Angle : ComplexToMagnitudeAngle  Output=Magnitude
  "Delta Pa PSS 133 " : powerlib/Machines/Generic Power System Stabilizer  Tsensor=15e-3  K=2.5*1.25  Twashout=1  Tleadlag1=[60e-3 1]  Tleadlag2=[0 0]  VSlimits=[-0.15 0.15]  Vinit=0  Plot_On=off  MagdB_On=on  FreqRange=logspace(-2,2,500)
      settings: SourceProductName=Simscape Power Systems  SourceProductBaseCode=PS
  "Delta w PSS (Kundur) 133 " : powerlib/Machines/Generic Power System Stabilizer  Tsensor=15e-3  K=30  Twashout=10  Tleadlag1=[50e-3 20e-3]  Tleadlag2=[3 5.4]  VSlimits=[-0.15 0.15]  Vinit=0  Plot_On=off  MagdB_On=on  FreqRange=logspace(-2,2,500)
      settings: SourceProductName=Simscape Power Systems  SourceProductBaseCode=PS
  MB-PSS  133 : powerlib/Machines/Multi-Band Power System Stabilizer  OperationMode=Simplified settings  Kg=1  GL=[0.1 10]  GI="[1  10]"  GH="[13  120]"  GLd=[66 66 9.4]  TcLF=[1.667 2 0 0 0 0 2 2.4 0 0 0 0 1 1]  GId=[66 66 47.6]  TcIF=[1 1 0.25 0.3 0 0 1 1 0.3 0.36 0 0 0 0]  GHd=[66 66 233]  TcHF="[0.01 0.012 0 0 0 0  0.012 0.0144 0 0 0 0 1 1]"  LIM=[.075 .15 .15 .15]  Plot_On=off  MagdB_On=off  FreqRange=logspace(-2,2,500)
      settings: SourceProductName=Simscape Power Systems  SourceProductBaseCode=PS
  Multiport Switch1 : MultiPortSwitch  Inputs=4  InputSameDT=on
  PSS model3 : Constant  Value=0
  PSS model4 : Constant
  Pref : Constant
  Real-Imag to Complex : RealImagToComplex
  STG 133 : powerlib/Machines/Steam Turbine and Governor  gentype=Tandem-compound (single mass)  reg1="[ 1  0.05    0 ]"  reg2="[ 0.001  0.15 ]"  reg3="[ -0.1  0.1  0  4.496 ]"  N=3600  turb1="[ 0  10   3.3   0.5   ]"  turb2="[   0   0.36    0.36   0.28   ]"  HA="[ 0.046  1.430  1.465   0.192 ]"  KA="[ 90.44  53.88  64.59   62.94  ]"  DA="[ 0.0115  0.3575  0.3663   0.0137  ]"  ini1=0.9  ini2=[0.779316,-31.4247]
      settings: SourceProductName=Simscape Power Systems  SourceProductBaseCode=PS
  Sum2 : Sum  SaturateOnIntegerOverflow=on  InputSameDT=on  OutDataTypeStr=Inherit: Same as first input
  Sum3 : Sum  Inputs=-+  SaturateOnIntegerOverflow=on  InputSameDT=on  OutDataTypeStr=Inherit: Same as first input
  Terminator1 : Terminator
  Terminator2 : Terminator
  Terminator3 : Terminator
  Vref01 : Constant
  wref : Constant
  A : PMIOPort  Side=Left
  B : PMIOPort  Port=2  Side=Left
  C : PMIOPort  Port=3  Side=Left
  tag scope: EFD133=global, Pa133=global, Pe133=global, Pm133=global, Q133=global, Vt133=global, d_theta133=global, pss133=global, theta133=global, w133=global
  wires:
  Bus Selector1/7 -> Real-Imag to Complex/2  "<Stator voltage  vq (pu)>"
  Bus Selector1/6 -> Real-Imag to Complex/1  "<Stator voltage  vd (pu)>"
  wref/1 -> STG 133/1
  Vref01/1 -> AC4A Excitation System 133/1
  Bus Selector1/4 -> [d_theta133], STG 133/4  "<Rotor angle deviation  d_theta (rad)>"
  133/1 -> Bus Selector1/1, [M133]
  Bus Selector1/1 -> [w133], STG 133/3  "<Rotor speed  wm  (pu)>"
  Bus Selector1/3 -> "Delta w PSS (Kundur) 133 "/1, MB-PSS  133/1  "<Rotor speed deviation  dw (pu)>"
  Real-Imag to Complex/1 -> Complex to Magnitude-Angle/1
  Complex to Magnitude-Angle/1 -> AC4A Excitation System 133/2, [Vt133]
  AC4A Excitation System 133/1 -> 133/2, [EFD133]
  Multiport Switch1/1 -> AC4A Excitation System 133/4, [pss133]
  Bus Selector1/5 -> [theta133]  "<Rotor mechanical angle  theta (deg)>"
  Bus Selector1/2 -> [Pe133]  "<Output active power   Peo (pu)>"
  Bus Selector1/8 -> AC4A Excitation System 133/3  "<Field current  ifd (pu)>"
  STG 133/4 -> [Pm133], 133/1
  Pref/1 -> STG 133/2
  Bus Selector1/9 -> [Q133]  "<Output reactive power  Qeo (pu)>"
  PSS model4/1 -> Sum2/2
  Sum2/1 -> Multiport Switch1/1
  [PSSmodel] -> Sum2/1
  PSS model3/1 -> Multiport Switch1/2
  Sum3/1 -> [Pa133], "Delta Pa PSS 133 "/1  "Pm-Pe"
  "Delta Pa PSS 133 "/1 -> Multiport Switch1/5
  "Delta w PSS (Kundur) 133 "/1 -> Multiport Switch1/4
  [Pm133] -> Sum3/2
  [Pe133] -> Sum3/1
  MB-PSS  133/1 -> Multiport Switch1/3
  STG 133/1 -> Terminator3/1
  STG 133/2 -> Terminator1/1
  STG 133/3 -> Terminator2/1
  connections:
  133/RConn1 -- A/RConn1
  133/RConn2 -- B/RConn1
  133/RConn3 -- C/RConn1

== system IEEE24bus/134 ==
  134 : powerlib/Machines/Synchronous Machine pu Standard  PresetModel=No  MechanicalLoad=Mechanical power Pm  ShowDetailedParameters=on  RotorType=Round  Units=per unit standard parameters  MeasurementBus=off  NominalParameters="[G_data(14,2)*1E6  G_data(14,3)*1E3  60]"  Reactances1=[G_data(14,6),G_data(14,8),G_data(14,10),G_data(14,7),G_data(14,12),G_data(14,14),G_data(14,5)]  Reactances2=[G_data(6,6),G_data(6,8),G_data(6,10),G_data(6,7),G_data(6,12),G_data(6,14),G_data(6,5)]  dAxisTimeConstants=Open-circuit  qAxisTimeConstants=Open-circuit  TimeConstants1="[G_data(6,9)  G_data(6,11)  G_data(6,13)  G_data(6,15)]"  TimeConstants2="[G_data(14,9)  G_data(14,11)  G_data(14,13)  G_data(14,15)]"  TimeConstants3="[  5.9  0.033  0.023  ]"  TimeConstants4=[ 8.0, 0.03, 0.3371, 0.0295 ]  TimeConstants5=[ 1.01, 0.053, 0.1 ]  TimeConstants6=[ 1.3201, 0.023, 1.0, 0.07 ]  TimeConstants7="[  1.01  0.053  0.051266  ]"  TimeConstants8=[ 1.3201, 0.0231, 0.3371, 0.0295 ]  StatorResistance=0  Mechanical="[ H134 0  4 ]"  PolePairs=4  InitialConditions=[0 -49.0871 0.832503 0.832503 0.832503 -10.6328 -130.633 109.367 2.39024]  SetSaturation=off  Saturation=[0.6404,0.7127,0.8441,0.9214,0.9956,1.082,1.19,1.316,1.457;0.7,0.7698,0.8872,0.9466,0.9969,1.046,1.1,1.151,1.201]  LoadFlowParameters=[1 3330000000 20000 0 0]  TsPowergui=0  TsBlock=-1  IterativeModel=Forward Euler  IterativeDiscreteModel=Trapezoidal non iterative  BusType=PV  Pref=G_data(14,2)*1e6  Qref=0  Qmin=-inf  Qmax=inf  PLF=0  QLF=0
      settings: SourceProductName=Simscape Power Systems
  AC4A Excitation System 134 : sps_avr/AC4A Excitation System  Tr=Exc(14,2)  KaTa="[Exc(14,3)   Exc(14,4)]"  VIminmax=[-10 10]  VRminmax=[-4.53 5.64]  TbTc="[Exc(14,5)  Exc(14,6)]"  Kc=0  v0=[1 2.3902]  TsBlock=0
      settings: SourceProductName=Simscape Power Systems  SourceProductBaseCode=PS
  Bus Selector1 : BusSelector  OutputSignals="Mechanical.Rotor speed  wm  (pu),Output active power   Peo (pu),Mechanical.Rotor speed deviation  dw (pu),Mechanical.Rotor angle deviation  d_theta (rad),Mechanical.Rotor mechanical angle  theta (deg),dq0 components.Stator voltage  vd (pu),dq0 components.Stator voltage  vq (pu),dq0 components.Field current  ifd (pu),Output reactive power  Qeo (pu)"
  Complex to Magnitude-Angle : ComplexToMagnitudeAngle  Output=Magnitude
  "Delta Pa PSS 134 " : powerlib/Machines/Generic Power System Stabilizer  Tsensor=15e-3  K=2.5*1.25  Twashout=1  Tleadlag1=[60e-3 1]  Tleadlag2=[0 0]  VSlimits=[-0.15 0.15]  Vinit=0  Plot_On=off  MagdB_On=on  FreqRange=logspace(-2,2,500)
      settings: SourceProductName=Simscape Power Systems  SourceProductBaseCode=PS
  "Delta w PSS (Kundur) 134 " : powerlib/Machines/Generic Power System Stabilizer  Tsensor=15e-3  K=30  Twashout=10  Tleadlag1=[50e-3 20e-3]  Tleadlag2=[3 5.4]  VSlimits=[-0.15 0.15]  Vinit=0  Plot_On=off  MagdB_On=on  FreqRange=logspace(-2,2,500)
      settings: SourceProductName=Simscape Power Systems  SourceProductBaseCode=PS
  MB-PSS  134 : powerlib/Machines/Multi-Band Power System Stabilizer  OperationMode=Simplified settings  Kg=1  GL=[0.1 10]  GI="[1  10]"  GH="[13  120]"  GLd=[66 66 9.4]  TcLF=[1.667 2 0 0 0 0 2 2.4 0 0 0 0 1 1]  GId=[66 66 47.6]  TcIF=[1 1 0.25 0.3 0 0 1 1 0.3 0.36 0 0 0 0]  GHd=[66 66 233]  TcHF="[0.01 0.012 0 0 0 0  0.012 0.0144 0 0 0 0 1 1]"  LIM=[.075 .15 .15 .15]  Plot_On=off  MagdB_On=off  FreqRange=logspace(-2,2,500)
      settings: SourceProductName=Simscape Power Systems  SourceProductBaseCode=PS
  Multiport Switch1 : MultiPortSwitch  Inputs=4  InputSameDT=on
  PSS model3 : Constant  Value=0
  PSS model4 : Constant
  Pref : Constant
  Real-Imag to Complex : RealImagToComplex
  STG 134 : powerlib/Machines/Steam Turbine and Governor  gentype=Tandem-compound (single mass)  reg1="[ 1  0.05    0 ]"  reg2="[ 0.001  0.15 ]"  reg3="[ -0.1  0.1  0  4.496 ]"  N=3600  turb1="[ 0  10   3.3   0.5   ]"  turb2="[   0   0.36    0.36   0.28   ]"  HA="[ 0.046  1.430  1.465   0.192 ]"  KA="[ 90.44  53.88  64.59   62.94  ]"  DA="[ 0.0115  0.3575  0.3663   0.0137  ]"  ini1=0.9  ini2=[0.779316,-31.4247]
      settings: SourceProductName=Simscape Power Systems  SourceProductBaseCode=PS
  Sum2 : Sum  SaturateOnIntegerOverflow=on  InputSameDT=on  OutDataTypeStr=Inherit: Same as first input
  Sum3 : Sum  Inputs=-+  SaturateOnIntegerOverflow=on  InputSameDT=on  OutDataTypeStr=Inherit: Same as first input
  Terminator1 : Terminator
  Terminator2 : Terminator
  Terminator3 : Terminator
  Vref01 : Constant
  wref : Constant
  A : PMIOPort  Side=Left
  B : PMIOPort  Port=2  Side=Left
  C : PMIOPort  Port=3  Side=Left
  tag scope: EFD134=global, Pa134=global, Pe134=global, Pm134=global, Q134=global, Vt134=global, d_theta134=global, pss134=global, theta134=global, w134=global
  wires:
  Bus Selector1/7 -> Real-Imag to Complex/2  "<Stator voltage  vq (pu)>"
  Bus Selector1/6 -> Real-Imag to Complex/1  "<Stator voltage  vd (pu)>"
  wref/1 -> STG 134/1
  Vref01/1 -> AC4A Excitation System 134/1
  Bus Selector1/4 -> [d_theta134], STG 134/4  "<Rotor angle deviation  d_theta (rad)>"
  134/1 -> Bus Selector1/1, [M134]
  Bus Selector1/1 -> [w134], STG 134/3  "<Rotor speed  wm  (pu)>"
  Bus Selector1/3 -> "Delta w PSS (Kundur) 134 "/1, MB-PSS  134/1  "<Rotor speed deviation  dw (pu)>"
  Real-Imag to Complex/1 -> Complex to Magnitude-Angle/1
  Complex to Magnitude-Angle/1 -> AC4A Excitation System 134/2, [Vt134]
  AC4A Excitation System 134/1 -> 134/2, [EFD134]
  Multiport Switch1/1 -> AC4A Excitation System 134/4, [pss134]
  Bus Selector1/5 -> [theta134]  "<Rotor mechanical angle  theta (deg)>"
  Bus Selector1/2 -> [Pe134]  "<Output active power   Peo (pu)>"
  Bus Selector1/8 -> AC4A Excitation System 134/3  "<Field current  ifd (pu)>"
  STG 134/4 -> [Pm134], 134/1
  Pref/1 -> STG 134/2
  Bus Selector1/9 -> [Q134]  "<Output reactive power  Qeo (pu)>"
  PSS model4/1 -> Sum2/2
  Sum2/1 -> Multiport Switch1/1
  [PSSmodel] -> Sum2/1
  PSS model3/1 -> Multiport Switch1/2
  Sum3/1 -> [Pa134], "Delta Pa PSS 134 "/1  "Pm-Pe"
  "Delta Pa PSS 134 "/1 -> Multiport Switch1/5
  "Delta w PSS (Kundur) 134 "/1 -> Multiport Switch1/4
  [Pm134] -> Sum3/2
  [Pe134] -> Sum3/1
  MB-PSS  134/1 -> Multiport Switch1/3
  STG 134/1 -> Terminator3/1
  STG 134/2 -> Terminator1/1
  STG 134/3 -> Terminator2/1
  connections:
  134/RConn1 -- A/RConn1
  134/RConn2 -- B/RConn1
  134/RConn3 -- C/RConn1

== system IEEE24bus/135 ==
  135 : powerlib/Machines/Synchronous Machine pu Standard  PresetModel=No  MechanicalLoad=Mechanical power Pm  ShowDetailedParameters=on  RotorType=Round  Units=per unit standard parameters  MeasurementBus=off  NominalParameters="[400*1E6  G_data(15,3)*1E3  60]"  Reactances1=[G_data(15,6),G_data(15,8),G_data(15,10),G_data(15,7),G_data(15,12),G_data(15,14),G_data(15,5)]  Reactances2=[G_data(6,6),G_data(6,8),G_data(6,10),G_data(6,7),G_data(6,12),G_data(6,14),G_data(6,5)]  dAxisTimeConstants=Open-circuit  qAxisTimeConstants=Open-circuit  TimeConstants1="[G_data(6,9)  G_data(6,11)  G_data(6,13)  G_data(6,15)]"  TimeConstants2="[G_data(15,9)  G_data(15,11)  G_data(15,13)  G_data(15,15)]"  TimeConstants3="[  5.9  0.033  0.023  ]"  TimeConstants4=[ 8.0, 0.03, 0.3371, 0.0295 ]  TimeConstants5=[ 1.01, 0.053, 0.1 ]  TimeConstants6=[ 1.3201, 0.023, 1.0, 0.07 ]  TimeConstants7="[  1.01  0.053  0.051266  ]"  TimeConstants8=[ 1.3201, 0.0231, 0.3371, 0.0295 ]  StatorResistance=0  Mechanical="[ H135 0  4 ]"  PolePairs=4  InitialConditions=[0 -49.0871 0.832503 0.832503 0.832503 -10.6328 -130.633 109.367 2.39024]  SetSaturation=off  Saturation=[0.6404,0.7127,0.8441,0.9214,0.9956,1.082,1.19,1.316,1.457;0.7,0.7698,0.8872,0.9466,0.9969,1.046,1.1,1.151,1.201]  LoadFlowParameters=[1 3330000000 20000 0 0]  TsPowergui=0  TsBlock=-1  IterativeModel=Forward Euler  IterativeDiscreteModel=Trapezoidal non iterative  BusType=PV  Pref=362.98*1e6  Qref=0  Qmin=-inf  Qmax=inf  PLF=0  QLF=0
      settings: SourceProductName=Simscape Power Systems
  AC4A Excitation System 135 : sps_avr/AC4A Excitation System  Tr=Exc(15,2)  KaTa="[Exc(15,3)   Exc(15,4)]"  VIminmax=[-10 10]  VRminmax=[-4.53 5.64]  TbTc="[Exc(15,5)  Exc(15,6)]"  Kc=0  v0=[1 2.3902]  TsBlock=0
      settings: SourceProductName=Simscape Power Systems  SourceProductBaseCode=PS
  Bus Selector1 : BusSelector  OutputSignals="Mechanical.Rotor speed  wm  (pu),Output active power   Peo (pu),Mechanical.Rotor speed deviation  dw (pu),Mechanical.Rotor angle deviation  d_theta (rad),Mechanical.Rotor mechanical angle  theta (deg),dq0 components.Stator voltage  vd (pu),dq0 components.Stator voltage  vq (pu),dq0 components.Field current  ifd (pu),Output reactive power  Qeo (pu)"
  Complex to Magnitude-Angle : ComplexToMagnitudeAngle  Output=Magnitude
  "Delta Pa PSS 135 " : powerlib/Machines/Generic Power System Stabilizer  Tsensor=15e-3  K=2.5*1.25  Twashout=1  Tleadlag1=[60e-3 1]  Tleadlag2=[0 0]  VSlimits=[-0.15 0.15]  Vinit=0  Plot_On=off  MagdB_On=on  FreqRange=logspace(-2,2,500)
      settings: SourceProductName=Simscape Power Systems  SourceProductBaseCode=PS
  "Delta w PSS (Kundur) 135 " : powerlib/Machines/Generic Power System Stabilizer  Tsensor=15e-3  K=30  Twashout=10  Tleadlag1=[50e-3 20e-3]  Tleadlag2=[3 5.4]  VSlimits=[-0.15 0.15]  Vinit=0  Plot_On=off  MagdB_On=on  FreqRange=logspace(-2,2,500)
      settings: SourceProductName=Simscape Power Systems  SourceProductBaseCode=PS
  MB-PSS  135 : powerlib/Machines/Multi-Band Power System Stabilizer  OperationMode=Simplified settings  Kg=1  GL=[0.1 10]  GI="[1  10]"  GH="[13  120]"  GLd=[66 66 9.4]  TcLF=[1.667 2 0 0 0 0 2 2.4 0 0 0 0 1 1]  GId=[66 66 47.6]  TcIF=[1 1 0.25 0.3 0 0 1 1 0.3 0.36 0 0 0 0]  GHd=[66 66 233]  TcHF="[0.01 0.012 0 0 0 0  0.012 0.0144 0 0 0 0 1 1]"  LIM=[.075 .15 .15 .15]  Plot_On=off  MagdB_On=off  FreqRange=logspace(-2,2,500)
      settings: SourceProductName=Simscape Power Systems  SourceProductBaseCode=PS
  Multiport Switch1 : MultiPortSwitch  Inputs=4  InputSameDT=on
  PSS model3 : Constant  Value=0
  PSS model4 : Constant
  Pref : Constant
  Real-Imag to Complex : RealImagToComplex
  STG 135 : powerlib/Machines/Steam Turbine and Governor  gentype=Tandem-compound (single mass)  reg1="[ 1  0.05    0 ]"  reg2="[ 0.001  0.15 ]"  reg3="[ -0.1  0.1  0  4.496 ]"  N=3600  turb1="[ 0  10   3.3   0.5   ]"  turb2="[   0   0.36    0.36   0.28   ]"  HA="[ 0.046  1.430  1.465   0.192 ]"  KA="[ 90.44  53.88  64.59   62.94  ]"  DA="[ 0.0115  0.3575  0.3663   0.0137  ]"  ini1=0.90  ini2=[0.779316,-31.4247]
      settings: SourceProductName=Simscape Power Systems  SourceProductBaseCode=PS
  Sum2 : Sum  SaturateOnIntegerOverflow=on  InputSameDT=on  OutDataTypeStr=Inherit: Same as first input
  Sum3 : Sum  Inputs=-+  SaturateOnIntegerOverflow=on  InputSameDT=on  OutDataTypeStr=Inherit: Same as first input
  Terminator1 : Terminator
  Terminator2 : Terminator
  Terminator3 : Terminator
  Vref01 : Constant
  wref : Constant
  A : PMIOPort  Side=Left
  B : PMIOPort  Port=2  Side=Left
  C : PMIOPort  Port=3  Side=Left
  tag scope: EFD135=global, Pa135=global, Pe135=global, Pm135=global, Q135=global, Vt135=global, d_theta135=global, pss135=global, theta135=global, w135=global
  wires:
  Bus Selector1/7 -> Real-Imag to Complex/2  "<Stator voltage  vq (pu)>"
  Bus Selector1/6 -> Real-Imag to Complex/1  "<Stator voltage  vd (pu)>"
  wref/1 -> STG 135/1
  Vref01/1 -> AC4A Excitation System 135/1
  Bus Selector1/4 -> [d_theta135], STG 135/4  "<Rotor angle deviation  d_theta (rad)>"
  135/1 -> Bus Selector1/1, [M135]
  Bus Selector1/1 -> [w135], STG 135/3  "<Rotor speed  wm  (pu)>"
  Bus Selector1/3 -> "Delta w PSS (Kundur) 135 "/1, MB-PSS  135/1  "<Rotor speed deviation  dw (pu)>"
  Real-Imag to Complex/1 -> Complex to Magnitude-Angle/1
  Complex to Magnitude-Angle/1 -> AC4A Excitation System 135/2, [Vt135]
  AC4A Excitation System 135/1 -> 135/2, [EFD135]
  Multiport Switch1/1 -> AC4A Excitation System 135/4, [pss135]
  Bus Selector1/5 -> [theta135]  "<Rotor mechanical angle  theta (deg)>"
  Bus Selector1/2 -> [Pe135]  "<Output active power   Peo (pu)>"
  Bus Selector1/8 -> AC4A Excitation System 135/3  "<Field current  ifd (pu)>"
  STG 135/4 -> [Pm135], 135/1
  Pref/1 -> STG 135/2
  Bus Selector1/9 -> [Q135]  "<Output reactive power  Qeo (pu)>"
  PSS model4/1 -> Sum2/2
  Sum2/1 -> Multiport Switch1/1
  [PSSmodel] -> Sum2/1
  PSS model3/1 -> Multiport Switch1/2
  Sum3/1 -> [Pa135], "Delta Pa PSS 135 "/1  "Pm-Pe"
  "Delta Pa PSS 135 "/1 -> Multiport Switch1/5
  "Delta w PSS (Kundur) 135 "/1 -> Multiport Switch1/4
  [Pm135] -> Sum3/2
  [Pe135] -> Sum3/1
  MB-PSS  135/1 -> Multiport Switch1/3
  STG 135/1 -> Terminator3/1
  STG 135/2 -> Terminator1/1
  STG 135/3 -> Terminator2/1
  connections:
  135/RConn1 -- A/RConn1
  135/RConn2 -- B/RConn1
  135/RConn3 -- C/RConn1
